simulink model "projectile_temp"  (Simulink 7.9)
settings: Solver=ode45  StartTime=0.0  StopTime=16  RelTol=1e-3
values from neighbouring files (symbols this model uses):
  CdC_m = 0.001731    [cmc_projectile_odegrads.m]    (also in cmc_projectile_odegrads2.m)
  g = 32.2    [cmc_projectile_odegrads.m]    (also in cmc_projectile_odegrads2.m)
  velx0 = cosd(theta)*vel0    [cmc_projectile_odegrads.m]    (also in cmc_projectile_odegrads2.m)
  vely0 = sind(theta)*vel0    [cmc_projectile_odegrads.m]    (also in cmc_projectile_odegrads2.m)
  x0 = 0    [Homework_3_ODEGRAD45.m]    (also in cmc_projectile_odegrads.m; cmc_projectile_odegrads2.m)
  y0 = 0.    (= 0)    [cmc_projectile_odegrads.m]    (also in cmc_projectile_odegrads2.m)
libraries: simulink x1
settings Model: Creator=cmc4177  LastModifiedBy=cmc4177

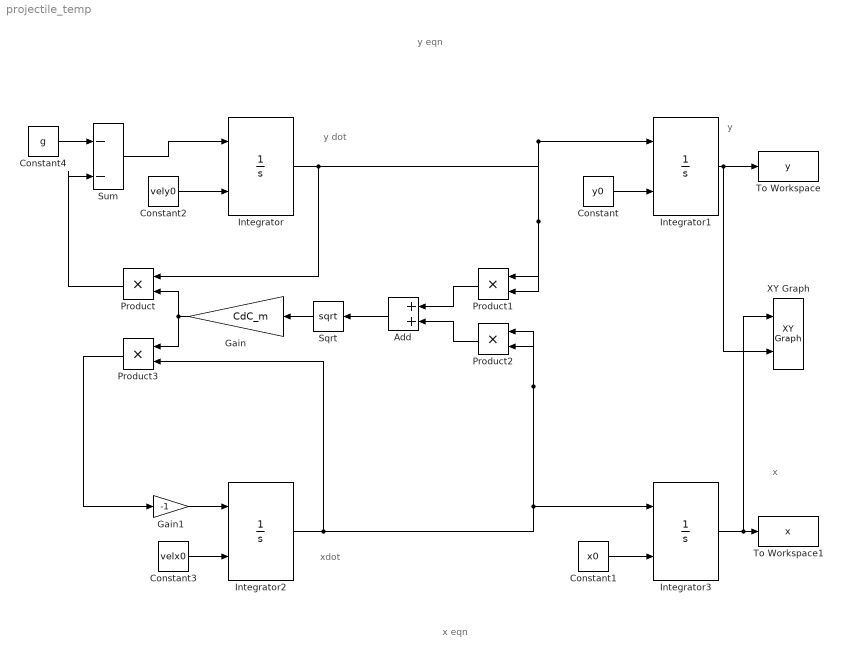
== system projectile_temp ==
  note: y eqn
  note: x eqn
  note: y dot
  note: y
  note: xdot
  note: x
  Add : Sum
  Constant : Constant  Value=y0
  Constant1 : Constant  Value=x0
  Constant2 : Constant  Value=vely0
  Constant3 : Constant  Value=velx0
  Constant4 : Constant  Value=g
  Gain : Gain  Gain=CdC_m
  Gain1 : Gain  Gain=-1
  Integrator{,1..3} (4 alike) : Integrator  InitialConditionSource=external
  Product{,1..3} (4 alike) : Product  RndMeth=Zero
  Sqrt : Sqrt  SaturateOnIntegerOverflow=on
  Sum : Sum  Inputs=--
  To Workspace : ToWorkspace  VariableName=y  SampleTime=-1
  To Workspace1 : ToWorkspace  VariableName=x  SampleTime=-1
  XY Graph : simulink/Sinks/XY Graph  xmin=-1  xmax=1  ymin=-1  ymax=1  st=-1
  wires:
  Integrator/1 -> Integrator1/1, Product1/1, Product1/2, Product/1
  Constant/1 -> Integrator1/2
  Constant1/1 -> Integrator3/2
  Constant3/1 -> Integrator2/2
  Constant2/1 -> Integrator/2
  Integrator2/1 -> Integrator3/1, Product2/2, Product2/1, Product3/2
  Product1/1 -> Add/1
  Product2/1 -> Add/2
  Add/1 -> Sqrt/1
  Sqrt/1 -> Gain/1
  Gain/1 -> Product/2, Product3/1
  Constant4/1 -> Sum/1
  Product/1 -> Sum/2
  Sum/1 -> Integrator/1
  Product3/1 -> Gain1/1
  Gain1/1 -> Integrator2/1
  Integrator1/1 -> XY Graph/2, To Workspace/1
  Integrator3/1 -> XY Graph/1, To Workspace1/1
